simulink model "ejemplo_planta_simulink"  (R2024b)
settings: Solver=VariableStepAuto  StartTime=0.0  StopTime=10.0  RelTol=1e-3
undefined symbols (not defined in the file or in its folder): a, b, K
settings Model: Creator=sergi  LastModifiedBy=sergi

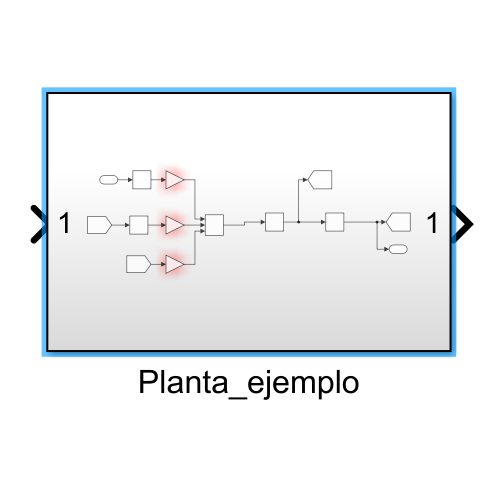
[thumbnail: Simulink's stored preview of the top-level diagram]
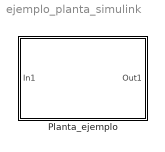
== system ejemplo_planta_simulink ==
  Planta_ejemplo : Subsystem

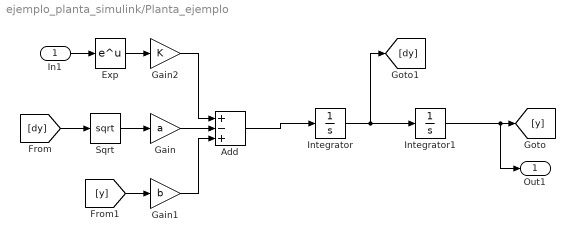
== system ejemplo_planta_simulink/Planta_ejemplo ==
  In1 : Inport
  Add : Sum  Inputs=+-+
  Exp : Math
  Gain : Gain  Gain=a
  Gain1 : Gain  Gain=b
  Gain2 : Gain  Gain=K
  Integrator : Integrator
  Integrator1 : Integrator
  Sqrt : Sqrt
  Out1 : Outport
  wires:
  Gain/1 -> Add/2
  Sqrt/1 -> Gain/1
  In1/1 -> Exp/1
  [dy] -> Sqrt/1
  Add/1 -> Integrator/1
  Integrator1/1 -> Out1/1, [y]
  Integrator/1 -> [dy], Integrator1/1
  Gain1/1 -> Add/3
  [y] -> Gain1/1
  Exp/1 -> Gain2/1
  Gain2/1 -> Add/1
